simulink model "twoMechanicalSystems"  (R2021a)
settings: Solver=VariableStepAuto  StartTime=0.0  StopTime=10.0  RelTol=1e-3
model workspace (MAT data in the model file):
  b = 4
  k1 = 5
  k2 = 3
  m1 = 2
  m2 = 2
undefined symbols (not defined in the file): DiscIntNeverNeededParam
settings Model: OrderedModelArguments=off  Creator=User  LastModifiedBy=User
settings OptimizationCC: DefaultParameterBehavior=Inlined  EnhancedBackFolding=on  PassReuseOutputArgsAs=Individual arguments  ZeroExternalMemoryAtStartup=off  ZeroInternalMemoryAtStartup=off  OptimizeBlockOrder=speed  DifferentSizesBufferReuse=on  OptimizationCustomize=off  EfficientTunableParamExpr=on
settings DebuggingCC: ParameterTunabilityLossMsg=error
settings SFSimCC: MATLABDynamicMemAlloc=off
settings RTWCC: SystemTargetFile=ert.tlc  TemplateMakefile=ert_default_tmf  Toolchain=MinGW64 | gmake (64-bit Windows)
settings CodeAppCC: ForceParamTrailComments=on  IgnoreCustomStorageClasses=off  OperatorAnnotations=on  SimulinkDataObjDesc=on  SFDataObjDesc=on  InsertBlockDesc=on
settings ERTTargetCC: TargetLangStandard=C99 (ISO)  GenerateSampleERTMain=on  InlinedParameterPlacement=NonHierarchical  ERTCustomFileTemplate=example_file_process.tlc

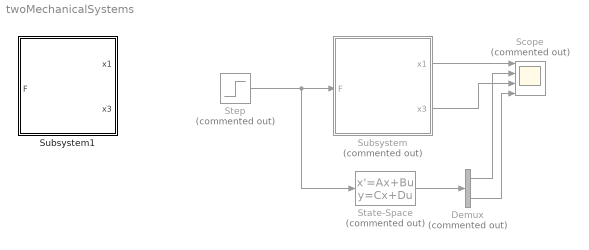
== system twoMechanicalSystems ==
  Demux : Demux  Commented=on  Outputs=2
  Scope : Scope  Commented=on  NumInputPorts=4
  State-Space : StateSpace  Commented=on  A=[0 1 0 0; (-k2/m2) (-b/m2) (k2/m2) (b/m2); 0 0 0 1; (k2/m1) (b/m1) (-(k2+k1)/m1) (-b/m1) ]  B=[0; 1; 0; 0;]  C=[1 0 0 0;0 0 1 0]  D=[0;0;]  InitialCondition=0
  Step : Step  Commented=on  SampleTime=0
  Subsystem : Subsystem  Commented=on  TreatAsAtomicUnit=on
  Subsystem1 : Subsystem  TreatAsAtomicUnit=on
  wires:
  Step/1 -> State-Space/1, Subsystem/1(F)
  State-Space/1 -> Demux/1
  Subsystem/1(x1) -> Scope/1
  Demux/1 -> Scope/2
  Subsystem/2(x3) -> Scope/3
  Demux/2 -> Scope/4

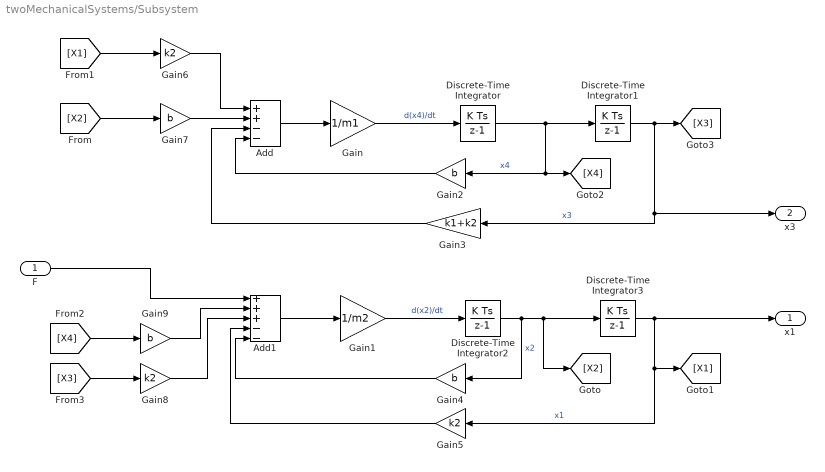
== system twoMechanicalSystems/Subsystem ==
  F : Inport
  Add : Sum  Inputs=++--
  Add1 : Sum  Inputs=+++--
  Discrete-Time Integrator{,1..3} (4 alike) : DiscreteIntegrator  SampleTime=-1  ICPrevOutput=DiscIntNeverNeededParam  ICPrevScaledInput=DiscIntNeverNeededParam
  Gain : Gain  Gain=1/m1
  Gain1 : Gain  Gain=1/m2
  Gain{2,4,7,9} (4 alike) : Gain  Gain=b
  Gain3 : Gain  Gain=k1+k2
  Gain5 : Gain  Gain=k2
  Gain6 : Gain  Gain=k2
  Gain8 : Gain  Gain=k2
  x1 : Outport
  x3 : Outport  Port=2
  wires:
  Discrete-Time Integrator/1 -> Discrete-Time Integrator1/1, [X4], Gain2/1  "x4"
  Discrete-Time Integrator2/1 -> Gain4/1, Discrete-Time Integrator3/1, [X2]  "x2"
  Discrete-Time Integrator3/1 -> x1/1, Gain5/1, [X1]  "x1"
  Add/1 -> Gain/1
  Gain6/1 -> Add/1
  Discrete-Time Integrator1/1 -> x3/1, Gain3/1, [X3]  "x3"
  Add1/1 -> Gain1/1
  Gain1/1 -> Discrete-Time Integrator2/1  "d(x2)/dt"
  [X3] -> Gain8/1
  Gain2/1 -> Add/4
  Gain3/1 -> Add/3
  Gain/1 -> Discrete-Time Integrator/1  "d(x4)/dt"
  Gain4/1 -> Add1/5
  Gain5/1 -> Add1/4
  [X1] -> Gain6/1
  Gain9/1 -> Add1/2
  Gain8/1 -> Add1/3
  [X4] -> Gain9/1
  Gain7/1 -> Add/2
  [X2] -> Gain7/1
  F/1 -> Add1/1

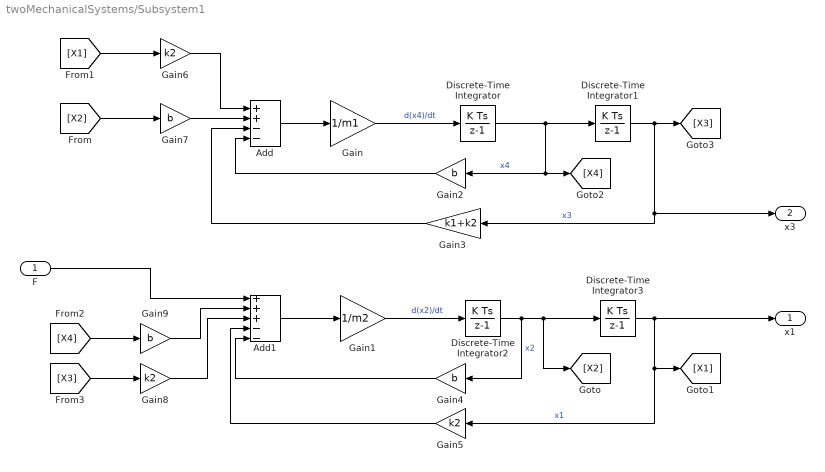
== system twoMechanicalSystems/Subsystem1 ==
  F : Inport
  Add : Sum  Inputs=++--
  Add1 : Sum  Inputs=+++--
  Discrete-Time Integrator{,1..3} (4 alike) : DiscreteIntegrator  SampleTime=-1  ICPrevOutput=DiscIntNeverNeededParam  ICPrevScaledInput=DiscIntNeverNeededParam
  Gain : Gain  Gain=1/m1
  Gain1 : Gain  Gain=1/m2
  Gain{2,4,7,9} (4 alike) : Gain  Gain=b
  Gain3 : Gain  Gain=k1+k2
  Gain5 : Gain  Gain=k2
  Gain6 : Gain  Gain=k2
  Gain8 : Gain  Gain=k2
  x1 : Outport
  x3 : Outport  Port=2
  wires:
  F/1 -> Add1/1
  [X2] -> Gain7/1
  Gain7/1 -> Add/2
  [X4] -> Gain9/1
  Gain8/1 -> Add1/3
  Gain9/1 -> Add1/2
  [X1] -> Gain6/1
  Gain5/1 -> Add1/4
  Gain4/1 -> Add1/5
  Gain/1 -> Discrete-Time Integrator/1  "d(x4)/dt"
  Gain3/1 -> Add/3
  Gain2/1 -> Add/4
  [X3] -> Gain8/1
  Gain1/1 -> Discrete-Time Integrator2/1  "d(x2)/dt"
  Add1/1 -> Gain1/1
  Discrete-Time Integrator1/1 -> [X3], Gain3/1, x3/1  "x3"
  Gain6/1 -> Add/1
  Add/1 -> Gain/1
  Discrete-Time Integrator3/1 -> [X1], Gain5/1, x1/1  "x1"
  Discrete-Time Integrator2/1 -> [X2], Discrete-Time Integrator3/1, Gain4/1  "x2"
  Discrete-Time Integrator/1 -> Gain2/1, [X4], Discrete-Time Integrator1/1  "x4"
